simulink library "dlbsBlockMatrixMultiply"  (R2025b)
settings: Solver=VariableStepAuto  StartTime=0.0  StopTime=10.0  RelTol=1e-3
libraries: dlbsBlockInsertGradientGF x2, dlbsBlockExtractGradientGF x1
settings Model: Creator=lt6037  LastModifiedBy=lt6037

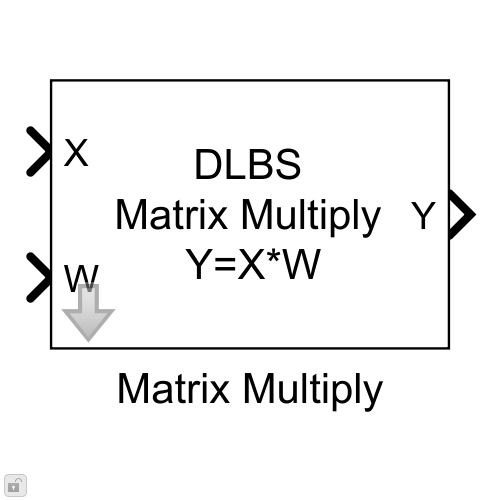
[thumbnail: Simulink's stored preview of the top-level diagram]
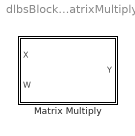
== system dlbsBlockMatrixMultiply ==
  Matrix Multiply : Subsystem
      mask help: Performs matrix multiplication between two compatible input matrices.
      mask Help: web("dlbsHelpBlockMatrixMultiply.html")
      mask Display: fprintf("DLBS\nMatrix Multiply\n Y=X*W")

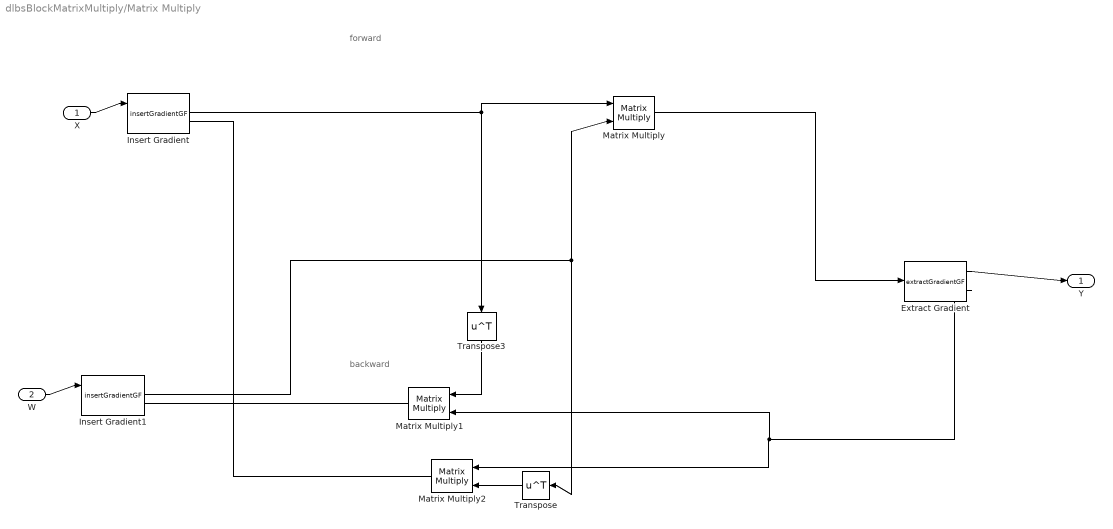
== system dlbsBlockMatrixMultiply/Matrix Multiply ==
  note: forward
  note: backward
  X : Inport
  W : Inport  Port=2
  Extract Gradient : dlbsBlockExtractGradientGF/extractGradientGF
  Insert Gradient : dlbsBlockInsertGradientGF/insertGradientGF
  Insert Gradient1 : dlbsBlockInsertGradientGF/insertGradientGF
  Matrix Multiply : Product  Multiplication=Matrix(*)
  Matrix Multiply1 : Product  Multiplication=Matrix(*)
  Matrix Multiply2 : Product  Multiplication=Matrix(*)
  Transpose : Math  Operator=transpose
  Transpose3 : Math  Operator=transpose
  Y : Outport
  wires:
  Matrix Multiply/1 -> Extract Gradient/1
  Insert Gradient1/1 -> Matrix Multiply/2, Transpose/1
  Transpose/1 -> Matrix Multiply2/2
  Transpose3/1 -> Matrix Multiply1/1
  Extract Gradient/2 -> Matrix Multiply2/1, Matrix Multiply1/2
  Insert Gradient/1 -> Matrix Multiply/1, Transpose3/1
  Matrix Multiply1/1 -> Insert Gradient1/2
  Matrix Multiply2/1 -> Insert Gradient/2
  X/1 -> Insert Gradient/1
  W/1 -> Insert Gradient1/1
  Extract Gradient/1 -> Y/1
